simulink library "inp"  (R2021b)
settings: Solver=VariableStepAuto  StartTime=0.0  StopTime=10.0  RelTol=1e-3
undefined symbols (not defined in the file): C_TASK_5MS_S, FALSE, KINP_AcoreReadyToSlp_flg_ovrdflg, KINP_AcoreReadyToSlp_flg_ovrdval, KINP_AllowMovThd_OTA_enum_ovrdflg, KINP_AllowMovThd_OTA_enum_ovrdval, KINP_APSAngleTarget_Deg_ovrdflg, KINP_APSAngleTarget_Deg_ovrdval, KINP_APSDecReq_mps2_ovrdflg, KINP_APSDecReq_mps2_ovrdval, KINP_APSDecReqA_flg_ovrdflg, KINP_APSDecReqA_flg_ovrdval, KINP_APSDFLL_cm_ovrdflg, KINP_APSDFLL_cm_ovrdval, KINP_APSDFLR_cm_ovrdflg, KINP_APSDFLR_cm_ovrdval, KINP_APSDRLL_cm_ovrdflg, KINP_APSDRLL_cm_ovrdval, KINP_APSDRLR_cm_ovrdflg, KINP_APSDRLR_cm_ovrdval, KINP_APSExitCondition_enum_ovrdflg, KINP_APSExitCondition_enum_ovrdval, KINP_APSHWVer_enum_ovrdflg, KINP_APSHWVer_enum_ovrdval, KINP_APSProgressPCT_pct_ovrdflg, KINP_APSProgressPCT_pct_ovrdval, KINP_APSReq_enum_ovrdflg, KINP_APSReq_enum_ovrdval, KINP_APSRQDisplay_enum_ovrdflg, KINP_APSRQDisplay_enum_ovrdval, KINP_APSRqEPASCtrl_flg_ovrdflg, KINP_APSRqEPASCtrl_flg_ovrdval, KINP_APSShiftPosnReq_enum_ovrdval, KINP_APSShiftPosnReq_enum_ovrflg, KINP_APSSpeedCMD_kph_ovrdval, KINP_APSSpeedCMD_kph_ovrflg, KINP_APSStaSystem_enum_ovrdflg, KINP_APSStaSystem_enum_ovrdval, KINP_APSSWVer_enum_ovrdflg, KINP_APSSWVer_enum_ovrdval, KINP_APSVMCReqA_flg_ovrdval, KINP_APSVMCReqA_flg_ovrflg, KINP_APSVRqEPASCtrl_flg_ovrdflg, KINP_APSVRqEPASCtrl_flg_ovrdval, KINP_AuxBattVolmV_mV_ovrdflg, KINP_AuxBattVolmV_mV_ovrdval, KINP_CAASSta_enum_ovrdflg, KINP_CAASSta_enum_ovrdval, KINP_CAASVMCReqA_flg_ovrdval, KINP_CAASVMCReqA_flg_ovrflg, KINP_Chime_enum_ovrdflg, KINP_Chime_enum_ovrdval, KINP_ClearDTCcmd_flg_ovrdflg, KINP_ClearDTCcmd_flg_ovrdval, KINP_EvccAplusPwrUpReq_flg_ovrdflg, KINP_EvccAplusPwrUpReq_flg_ovrdval, KINP_LFID_raw_ovrdval, KINP_LFID_raw_ovrflg, KINP_LRID_raw_ovrdval, KINP_MemOffsetAccX_raw16_ovrdflg ... (+118)
libraries: FVT_lib x595, hcu_lib x1
(part 26 of 27)

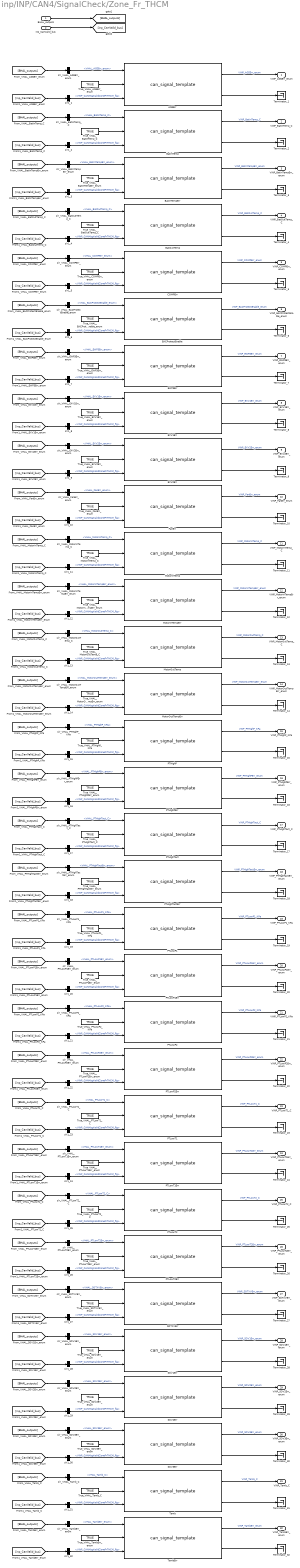
== system inp/INP/CAN4/SignalCheck/Zone_Fr_THCM ==
  BHAL_outputs : Inport
  inp_CanValid_bus : Inport  Port=2
  AGSErr : FVT_lib/inp/can_signal_template  SystemSampleTime=-1  VariantActivationTime=update diagram  Latency=0  AutoFrameSizeCalculation=off
      link override defval: Value=KINP_AGSErr_enum_defval
      link override fftdec: Value=KINP_AGSErr_enum_fftdec
      link override fftinc: Value=KINP_AGSErr_enum_fftinc
      link override fftlim: Value=KINP_AGSErr_enum_fftlim
      link override invalid: Value=KINP_AGSErr_enum_invalid
      link override ovrdflg: Value=KINP_AGSErr_enum_ovrdflg
      link override ovrdval: Value=KINP_AGSErr_enum_ovrdval
      link override setvalid: Value=KINP_AGSErr_enum_setvalid
      link override srvcflg: Value=KINP_AGSErr_enum_srvcflg
      link override srvcval: Value=KINP_AGSErr_enum_srvcval
  BatInTemp : FVT_lib/inp/can_signal_template  SystemSampleTime=-1  VariantActivationTime=update diagram  Latency=0  AutoFrameSizeCalculation=off
      link override defval: Value=KINP_BatInTemp_C_defval
      link override fftdec: Value=KINP_BatInTemp_C_fftdec
      link override fftinc: Value=KINP_BatInTemp_C_fftinc
      link override fftlim: Value=KINP_BatInTemp_C_fftlim
      link override invalid: Value=KINP_BatInTemp_C_invalid
      link override ovrdflg: Value=KINP_BatInTemp_C_ovrdflg
      link override ovrdval: Value=KINP_BatInTemp_C_ovrdval
      link override setvalid: Value=KINP_BatInTemp_C_setvalid
      link override srvcflg: Value=KINP_BatInTemp_C_srvcflg
      link override srvcval: Value=KINP_BatInTemp_C_srvcval
  BatInTempErr : FVT_lib/inp/can_signal_template  SystemSampleTime=-1  VariantActivationTime=update diagram  Latency=0  AutoFrameSizeCalculation=off
      link override defval: Value=KINP_BatInTempErr_enum_defval
      link override fftdec: Value=KINP_BatInTempErr_enum_fftdec
      link override fftinc: Value=KINP_BatInTempErr_enum_fftinc
      link override fftlim: Value=KINP_BatInTempErr_enum_fftlim
      link override invalid: Value=KINP_BatInTempErr_enum_invalid
      link override ovrdflg: Value=KINP_BatInTempErr_enum_ovrdflg
      link override ovrdval: Value=KINP_BatInTempErr_enum_ovrdval
      link override setvalid: Value=KINP_BatInTempErr_enum_setvalid
      link override srvcflg: Value=KINP_BatInTempErr_enum_srvcflg
      link override srvcval: Value=KINP_BatInTempErr_enum_srvcval
  BatOutTemp : FVT_lib/inp/can_signal_template  SystemSampleTime=-1  VariantActivationTime=update diagram  Latency=0  AutoFrameSizeCalculation=off
      link override defval: Value=KINP_BatOutTemp_C_defval
      link override fftdec: Value=KINP_BatOutTemp_C_fftdec
      link override fftinc: Value=KINP_BatOutTemp_C_fftinc
      link override fftlim: Value=KINP_BatOutTemp_C_fftlim
      link override invalid: Value=KINP_BatOutTemp_C_invalid
      link override ovrdflg: Value=KINP_BatOutTemp_C_ovrdflg
      link override ovrdval: Value=KINP_BatOutTemp_C_ovrdval
      link override setvalid: Value=KINP_BatOutTemp_C_setvalid
      link override srvcflg: Value=KINP_BatOutTemp_C_srvcflg
      link override srvcval: Value=KINP_BatOutTemp_C_srvcval
  COMPErr : FVT_lib/inp/can_signal_template  SystemSampleTime=-1  VariantActivationTime=update diagram  Latency=0  AutoFrameSizeCalculation=off
      link override defval: Value=KINP_COMPErr_enum_defval
      link override fftdec: Value=KINP_COMPErr_enum_fftdec
      link override fftinc: Value=KINP_COMPErr_enum_fftinc
      link override fftlim: Value=KINP_COMPErr_enum_fftlim
      link override invalid: Value=KINP_COMPErr_enum_invalid
      link override ovrdflg: Value=KINP_COMPErr_enum_ovrdflg
      link override ovrdval: Value=KINP_COMPErr_enum_ovrdval
      link override setvalid: Value=KINP_COMPErr_enum_setvalid
      link override srvcflg: Value=KINP_COMPErr_enum_srvcflg
      link override srvcval: Value=KINP_COMPErr_enum_srvcval
  EACProtectEnable : FVT_lib/inp/can_signal_template  SystemSampleTime=-1  VariantActivationTime=update diagram  Latency=0  AutoFrameSizeCalculation=off
      link override defval: Value=KINP_EACProtectEnable_enum_defval
      link override fftdec: Value=KINP_EACProtectEnable_enum_fftdec
      link override fftinc: Value=KINP_EACProtectEnable_enum_fftinc
      link override fftlim: Value=KINP_EACProtectEnable_enum_fftlim
      link override invalid: Value=KINP_EACProtectEnable_enum_invalid
      link override ovrdflg: Value=KINP_EACProtectEnable_enum_ovrdflg
      link override ovrdval: Value=KINP_EACProtectEnable_enum_ovrdval
      link override setvalid: Value=KINP_EACProtectEnable_enum_setvalid
      link override srvcflg: Value=KINP_EACProtectEnable_enum_srvcflg
      link override srvcval: Value=KINP_EACProtectEnable_enum_srvcval
  EWP3Err : FVT_lib/inp/can_signal_template  SystemSampleTime=-1  VariantActivationTime=update diagram  Latency=0  AutoFrameSizeCalculation=off
      link override defval: Value=KINP_EWP3Err_enum_defval
      link override fftdec: Value=KINP_EWP3Err_enum_fftdec
      link override fftinc: Value=KINP_EWP3Err_enum_fftinc
      link override fftlim: Value=KINP_EWP3Err_enum_fftlim
      link override invalid: Value=KINP_EWP3Err_enum_invalid
      link override ovrdflg: Value=KINP_EWP3Err_enum_ovrdflg
      link override ovrdval: Value=KINP_EWP3Err_enum_ovrdval
      link override setvalid: Value=KINP_EWP3Err_enum_setvalid
      link override srvcflg: Value=KINP_EWP3Err_enum_srvcflg
      link override srvcval: Value=KINP_EWP3Err_enum_srvcval
  EXV1Err : FVT_lib/inp/can_signal_template  SystemSampleTime=-1  VariantActivationTime=update diagram  Latency=0  AutoFrameSizeCalculation=off
      link override defval: Value=KINP_EXV1Err_enum_defval
      link override fftdec: Value=KINP_EXV1Err_enum_fftdec
      link override fftinc: Value=KINP_EXV1Err_enum_fftinc
      link override fftlim: Value=KINP_EXV1Err_enum_fftlim
      link override invalid: Value=KINP_EXV1Err_enum_invalid
      link override ovrdflg: Value=KINP_EXV1Err_enum_ovrdflg
      link override ovrdval: Value=KINP_EXV1Err_enum_ovrdval
      link override setvalid: Value=KINP_EXV1Err_enum_setvalid
      link override srvcflg: Value=KINP_EXV1Err_enum_srvcflg
      link override srvcval: Value=KINP_EXV1Err_enum_srvcval
  EXV2Err : FVT_lib/inp/can_signal_template  SystemSampleTime=-1  VariantActivationTime=update diagram  Latency=0  AutoFrameSizeCalculation=off
      link override defval: Value=KINP_EXV2Err_enum_defval
      link override fftdec: Value=KINP_EXV2Err_enum_fftdec
      link override fftinc: Value=KINP_EXV2Err_enum_fftinc
      link override fftlim: Value=KINP_EXV2Err_enum_fftlim
      link override invalid: Value=KINP_EXV2Err_enum_invalid
      link override ovrdflg: Value=KINP_EXV2Err_enum_ovrdflg
      link override ovrdval: Value=KINP_EXV2Err_enum_ovrdval
      link override setvalid: Value=KINP_EXV2Err_enum_setvalid
      link override srvcflg: Value=KINP_EXV2Err_enum_srvcflg
      link override srvcval: Value=KINP_EXV2Err_enum_srvcval
  FanErr : FVT_lib/inp/can_signal_template  SystemSampleTime=-1  VariantActivationTime=update diagram  Latency=0  AutoFrameSizeCalculation=off
      link override defval: Value=KINP_FanErr_enum_defval
      link override fftdec: Value=KINP_FanErr_enum_fftdec
      link override fftinc: Value=KINP_FanErr_enum_fftinc
      link override fftlim: Value=KINP_FanErr_enum_fftlim
      link override invalid: Value=KINP_FanErr_enum_invalid
      link override ovrdflg: Value=KINP_FanErr_enum_ovrdflg
      link override ovrdval: Value=KINP_FanErr_enum_ovrdval
      link override setvalid: Value=KINP_FanErr_enum_setvalid
      link override srvcflg: Value=KINP_FanErr_enum_srvcflg
      link override srvcval: Value=KINP_FanErr_enum_srvcval
  MotorInTemp : FVT_lib/inp/can_signal_template  SystemSampleTime=-1  VariantActivationTime=update diagram  Latency=0  AutoFrameSizeCalculation=off
      link override defval: Value=KINP_MotorInTemp_C_defval
      link override fftdec: Value=KINP_MotorInTemp_C_fftdec
      link override fftinc: Value=KINP_MotorInTemp_C_fftinc
      link override fftlim: Value=KINP_MotorInTemp_C_fftlim
      link override invalid: Value=KINP_MotorInTemp_C_invalid
      link override ovrdflg: Value=KINP_MotorInTemp_C_ovrdflg
      link override ovrdval: Value=KINP_MotorInTemp_C_ovrdval
      link override setvalid: Value=KINP_MotorInTemp_C_setvalid
      link override srvcflg: Value=KINP_MotorInTemp_C_srvcflg
      link override srvcval: Value=KINP_MotorInTemp_C_srvcval
  MotorInTempErr : FVT_lib/inp/can_signal_template  SystemSampleTime=-1  VariantActivationTime=update diagram  Latency=0  AutoFrameSizeCalculation=off
      link override defval: Value=KINP_MotorInTempErr_enum_defval
      link override fftdec: Value=KINP_MotorInTempErr_enum_fftdec
      link override fftinc: Value=KINP_MotorInTempErr_enum_fftinc
      link override fftlim: Value=KINP_MotorInTempErr_enum_fftlim
      link override invalid: Value=KINP_MotorInTempErr_enum_invalid
      link override ovrdflg: Value=KINP_MotorInTempErr_enum_ovrdflg
      link override ovrdval: Value=KINP_MotorInTempErr_enum_ovrdval
      link override setvalid: Value=KINP_MotorInTempErr_enum_setvalid
      link override srvcflg: Value=KINP_MotorInTempErr_enum_srvcflg
      link override srvcval: Value=KINP_MotorInTempErr_enum_srvcval
  MotorOutTemp : FVT_lib/inp/can_signal_template  SystemSampleTime=-1  VariantActivationTime=update diagram  Latency=0  AutoFrameSizeCalculation=off
      link override defval: Value=KINP_MotorOutTemp_C_defval
      link override fftdec: Value=KINP_MotorOutTemp_C_fftdec
      link override fftinc: Value=KINP_MotorOutTemp_C_fftinc
      link override fftlim: Value=KINP_MotorOutTemp_C_fftlim
      link override invalid: Value=KINP_MotorOutTemp_C_invalid
      link override ovrdflg: Value=KINP_MotorOutTemp_C_ovrdflg
      link override ovrdval: Value=KINP_MotorOutTemp_C_ovrdval
      link override setvalid: Value=KINP_MotorOutTemp_C_setvalid
      link override srvcflg: Value=KINP_MotorOutTemp_C_srvcflg
      link override srvcval: Value=KINP_MotorOutTemp_C_srvcval
  MotorOutTempErr : FVT_lib/inp/can_signal_template  SystemSampleTime=-1  VariantActivationTime=update diagram  Latency=0  AutoFrameSizeCalculation=off
      link override defval: Value=KINP_MotorOutTempErr_enum_defval
      link override fftdec: Value=KINP_MotorOutTempErr_enum_fftdec
      link override fftinc: Value=KINP_MotorOutTempErr_enum_fftinc
      link override fftlim: Value=KINP_MotorOutTempErr_enum_fftlim
      link override invalid: Value=KINP_MotorOutTempErr_enum_invalid
      link override ovrdflg: Value=KINP_MotorOutTempErr_enum_ovrdflg
      link override ovrdval: Value=KINP_MotorOutTempErr_enum_ovrdval
      link override setvalid: Value=KINP_MotorOutTempErr_enum_setvalid
      link override srvcflg: Value=KINP_MotorOutTempErr_enum_srvcflg
      link override srvcval: Value=KINP_MotorOutTempErr_enum_srvcval
  PTHighP : FVT_lib/inp/can_signal_template  SystemSampleTime=-1  VariantActivationTime=update diagram  Latency=0  AutoFrameSizeCalculation=off
      link override defval: Value=KINP_PTHighP_KPa_defval
      link override fftdec: Value=KINP_PTHighP_KPa_fftdec
      link override fftinc: Value=KINP_PTHighP_KPa_fftinc
      link override fftlim: Value=KINP_PTHighP_KPa_fftlim
      link override invalid: Value=KINP_PTHighP_KPa_invalid
      link override ovrdflg: Value=KINP_PTHighP_KPa_ovrdflg
      link override ovrdval: Value=KINP_PTHighP_KPa_ovrdval
      link override setvalid: Value=KINP_PTHighP_KPa_setvalid
      link override srvcflg: Value=KINP_PTHighP_KPa_srvcflg
      link override srvcval: Value=KINP_PTHighP_KPa_srvcval
  PTHighPErr : FVT_lib/inp/can_signal_template  SystemSampleTime=-1  VariantActivationTime=update diagram  Latency=0  AutoFrameSizeCalculation=off
      link override defval: Value=KINP_PTHighPErr_enum_defval
      link override fftdec: Value=KINP_PTHighPErr_enum_fftdec
      link override fftinc: Value=KINP_PTHighPErr_enum_fftinc
      link override fftlim: Value=KINP_PTHighPErr_enum_fftlim
      link override invalid: Value=KINP_PTHighPErr_enum_invalid
      link override ovrdflg: Value=KINP_PTHighPErr_enum_ovrdflg
      link override ovrdval: Value=KINP_PTHighPErr_enum_ovrdval
      link override setvalid: Value=KINP_PTHighPErr_enum_setvalid
      link override srvcflg: Value=KINP_PTHighPErr_enum_srvcflg
      link override srvcval: Value=KINP_PTHighPErr_enum_srvcval
  PTHighTact : FVT_lib/inp/can_signal_template  SystemSampleTime=-1  VariantActivationTime=update diagram  Latency=0  AutoFrameSizeCalculation=off
      link override defval: Value=KINP_PTHighTact_C_defval
      link override fftdec: Value=KINP_PTHighTact_C_fftdec
      link override fftinc: Value=KINP_PTHighTact_C_fftinc
      link override fftlim: Value=KINP_PTHighTact_C_fftlim
      link override invalid: Value=KINP_PTHighTact_C_invalid
      link override ovrdflg: Value=KINP_PTHighTact_C_ovrdflg
      link override ovrdval: Value=KINP_PTHighTact_C_ovrdval
      link override setvalid: Value=KINP_PTHighTact_C_setvalid
      link override srvcflg: Value=KINP_PTHighTact_C_srvcflg
      link override srvcval: Value=KINP_PTHighTact_C_srvcval
  PTHighTactErr : FVT_lib/inp/can_signal_template  SystemSampleTime=-1  VariantActivationTime=update diagram  Latency=0  AutoFrameSizeCalculation=off
      link override defval: Value=KINP_PTHighTactErr_enum_defval
      link override fftdec: Value=KINP_PTHighTactErr_enum_fftdec
      link override fftinc: Value=KINP_PTHighTactErr_enum_fftinc
      link override fftlim: Value=KINP_PTHighTactErr_enum_fftlim
      link override invalid: Value=KINP_PTHighTactErr_enum_invalid
      link override ovrdflg: Value=KINP_PTHighTactErr_enum_ovrdflg
      link override ovrdval: Value=KINP_PTHighTactErr_enum_ovrdval
      link override setvalid: Value=KINP_PTHighTactErr_enum_setvalid
      link override srvcflg: Value=KINP_PTHighTactErr_enum_srvcflg
      link override srvcval: Value=KINP_PTHighTactErr_enum_srvcval
  PTLowP1 : FVT_lib/inp/can_signal_template  SystemSampleTime=-1  VariantActivationTime=update diagram  Latency=0  AutoFrameSizeCalculation=off
      link override defval: Value=KINP_PTLowP1_KPa_defval
      link override fftdec: Value=KINP_PTLowP1_KPa_fftdec
      link override fftinc: Value=KINP_PTLowP1_KPa_fftinc
      link override fftlim: Value=KINP_PTLowP1_KPa_fftlim
      link override invalid: Value=KINP_PTLowP1_KPa_invalid
      link override ovrdflg: Value=KINP_PTLowP1_KPa_ovrdflg
      link override ovrdval: Value=KINP_PTLowP1_KPa_ovrdval
      link override setvalid: Value=KINP_PTLowP1_KPa_setvalid
      link override srvcflg: Value=KINP_PTLowP1_KPa_srvcflg
      link override srvcval: Value=KINP_PTLowP1_KPa_srvcval
  PTLowP1Err : FVT_lib/inp/can_signal_template  SystemSampleTime=-1  VariantActivationTime=update diagram  Latency=0  AutoFrameSizeCalculation=off
      link override defval: Value=KINP_PTLowP1Err_enum_defval
      link override fftdec: Value=KINP_PTLowP1Err_enum_fftdec
      link override fftinc: Value=KINP_PTLowP1Err_enum_fftinc
      link override fftlim: Value=KINP_PTLowP1Err_enum_fftlim
      link override invalid: Value=KINP_PTLowP1Err_enum_invalid
      link override ovrdflg: Value=KINP_PTLowP1Err_enum_ovrdflg
      link override ovrdval: Value=KINP_PTLowP1Err_enum_ovrdval
      link override setvalid: Value=KINP_PTLowP1Err_enum_setvalid
      link override srvcflg: Value=KINP_PTLowP1Err_enum_srvcflg
      link override srvcval: Value=KINP_PTLowP1Err_enum_srvcval
  PTLowP2 : FVT_lib/inp/can_signal_template  SystemSampleTime=-1  VariantActivationTime=update diagram  Latency=0  AutoFrameSizeCalculation=off
      link override defval: Value=KINP_PTLowP2_KPa_defval
      link override fftdec: Value=KINP_PTLowP2_KPa_fftdec
      link override fftinc: Value=KINP_PTLowP2_KPa_fftinc
      link override fftlim: Value=KINP_PTLowP2_KPa_fftlim
      link override invalid: Value=KINP_PTLowP2_KPa_invalid
      link override ovrdflg: Value=KINP_PTLowP2_KPa_ovrdflg
      link override ovrdval: Value=KINP_PTLowP2_KPa_ovrdval
      link override setvalid: Value=KINP_PTLowP2_KPa_setvalid
      link override srvcflg: Value=KINP_PTLowP2_KPa_srvcflg
      link override srvcval: Value=KINP_PTLowP2_KPa_srvcval
  PTLowP2Err : FVT_lib/inp/can_signal_template  SystemSampleTime=-1  VariantActivationTime=update diagram  Latency=0  AutoFrameSizeCalculation=off
      link override defval: Value=KINP_PTLowP2Err_enum_defval
      link override fftdec: Value=KINP_PTLowP2Err_enum_fftdec
      link override fftinc: Value=KINP_PTLowP2Err_enum_fftinc
      link override fftlim: Value=KINP_PTLowP2Err_enum_fftlim
      link override invalid: Value=KINP_PTLowP2Err_enum_invalid
      link override ovrdflg: Value=KINP_PTLowP2Err_enum_ovrdflg
      link override ovrdval: Value=KINP_PTLowP2Err_enum_ovrdval
      link override setvalid: Value=KINP_PTLowP2Err_enum_setvalid
      link override srvcflg: Value=KINP_PTLowP2Err_enum_srvcflg
      link override srvcval: Value=KINP_PTLowP2Err_enum_srvcval
  PTLowT1 : FVT_lib/inp/can_signal_template  SystemSampleTime=-1  VariantActivationTime=update diagram  Latency=0  AutoFrameSizeCalculation=off
      link override defval: Value=KINP_PTLowT1_C_defval
      link override fftdec: Value=KINP_PTLowT1_C_fftdec
      link override fftinc: Value=KINP_PTLowT1_C_fftinc
      link override fftlim: Value=KINP_PTLowT1_C_fftlim
      link override invalid: Value=KINP_PTLowT1_C_invalid
      link override ovrdflg: Value=KINP_PTLowT1_C_ovrdflg
      link override ovrdval: Value=KINP_PTLowT1_C_ovrdval
      link override setvalid: Value=KINP_PTLowT1_C_setvalid
      link override srvcflg: Value=KINP_PTLowT1_C_srvcflg
      link override srvcval: Value=KINP_PTLowT1_C_srvcval
  PTLowT1Err : FVT_lib/inp/can_signal_template  SystemSampleTime=-1  VariantActivationTime=update diagram  Latency=0  AutoFrameSizeCalculation=off
      link override defval: Value=KINP_PTLowT1Err_enum_defval
      link override fftdec: Value=KINP_PTLowT1Err_enum_fftdec
      link override fftinc: Value=KINP_PTLowT1Err_enum_fftinc
      link override fftlim: Value=KINP_PTLowT1Err_enum_fftlim
      link override invalid: Value=KINP_PTLowT1Err_enum_invalid
      link override ovrdflg: Value=KINP_PTLowT1Err_enum_ovrdflg
      link override ovrdval: Value=KINP_PTLowT1Err_enum_ovrdval
      link override setvalid: Value=KINP_PTLowT1Err_enum_setvalid
      link override srvcflg: Value=KINP_PTLowT1Err_enum_srvcflg
      link override srvcval: Value=KINP_PTLowT1Err_enum_srvcval
  PTLowT2 : FVT_lib/inp/can_signal_template  SystemSampleTime=-1  VariantActivationTime=update diagram  Latency=0  AutoFrameSizeCalculation=off
      link override defval: Value=KINP_PTLowT2_C_defval
      link override fftdec: Value=KINP_PTLowT2_C_fftdec
      link override fftinc: Value=KINP_PTLowT2_C_fftinc
      link override fftlim: Value=KINP_PTLowT2_C_fftlim
      link override invalid: Value=KINP_PTLowT2_C_invalid
      link override ovrdflg: Value=KINP_PTLowT2_C_ovrdflg
      link override ovrdval: Value=KINP_PTLowT2_C_ovrdval
      link override setvalid: Value=KINP_PTLowT2_C_setvalid
      link override srvcflg: Value=KINP_PTLowT2_C_srvcflg
      link override srvcval: Value=KINP_PTLowT2_C_srvcval
  PTLowT2Err : FVT_lib/inp/can_signal_template  SystemSampleTime=-1  VariantActivationTime=update diagram  Latency=0  AutoFrameSizeCalculation=off
      link override defval: Value=KINP_PTLowT2Err_enum_defval
      link override fftdec: Value=KINP_PTLowT2Err_enum_fftdec
      link override fftinc: Value=KINP_PTLowT2Err_enum_fftinc
      link override fftlim: Value=KINP_PTLowT2Err_enum_fftlim
      link override invalid: Value=KINP_PTLowT2Err_enum_invalid
      link override ovrdflg: Value=KINP_PTLowT2Err_enum_ovrdflg
      link override ovrdval: Value=KINP_PTLowT2Err_enum_ovrdval
      link override setvalid: Value=KINP_PTLowT2Err_enum_setvalid
      link override srvcflg: Value=KINP_PTLowT2Err_enum_srvcflg
      link override srvcval: Value=KINP_PTLowT2Err_enum_srvcval
  SOTXVErr : FVT_lib/inp/can_signal_template  SystemSampleTime=-1  VariantActivationTime=update diagram  Latency=0  AutoFrameSizeCalculation=off
      link override defval: Value=KINP_SOTXVErr_enum_defval
      link override fftdec: Value=KINP_SOTXVErr_enum_fftdec
      link override fftinc: Value=KINP_SOTXVErr_enum_fftinc
      link override fftlim: Value=KINP_SOTXVErr_enum_fftlim
      link override invalid: Value=KINP_SOTXVErr_enum_invalid
      link override ovrdflg: Value=KINP_SOTXVErr_enum_ovrdflg
      link override ovrdval: Value=KINP_SOTXVErr_enum_ovrdval
      link override setvalid: Value=KINP_SOTXVErr_enum_setvalid
      link override srvcflg: Value=KINP_SOTXVErr_enum_srvcflg
      link override srvcval: Value=KINP_SOTXVErr_enum_srvcval
  SOV1Err : FVT_lib/inp/can_signal_template  SystemSampleTime=-1  VariantActivationTime=update diagram  Latency=0  AutoFrameSizeCalculation=off
      link override defval: Value=KINP_SOV1Err_enum_defval
      link override fftdec: Value=KINP_SOV1Err_enum_fftdec
      link override fftinc: Value=KINP_SOV1Err_enum_fftinc
      link override fftlim: Value=KINP_SOV1Err_enum_fftlim
      link override invalid: Value=KINP_SOV1Err_enum_invalid
      link override ovrdflg: Value=KINP_SOV1Err_enum_ovrdflg
      link override ovrdval: Value=KINP_SOV1Err_enum_ovrdval
      link override setvalid: Value=KINP_SOV1Err_enum_setvalid
      link override srvcflg: Value=KINP_SOV1Err_enum_srvcflg
      link override srvcval: Value=KINP_SOV1Err_enum_srvcval
  SOV2Err : FVT_lib/inp/can_signal_template  SystemSampleTime=-1  VariantActivationTime=update diagram  Latency=0  AutoFrameSizeCalculation=off
      link override defval: Value=KINP_SOV2Err_enum_defval
      link override fftdec: Value=KINP_SOV2Err_enum_fftdec
      link override fftinc: Value=KINP_SOV2Err_enum_fftinc
      link override fftlim: Value=KINP_SOV2Err_enum_fftlim
      link override invalid: Value=KINP_SOV2Err_enum_invalid
      link override ovrdflg: Value=KINP_SOV2Err_enum_ovrdflg
      link override ovrdval: Value=KINP_SOV2Err_enum_ovrdval
      link override setvalid: Value=KINP_SOV2Err_enum_setvalid
      link override srvcflg: Value=KINP_SOV2Err_enum_srvcflg
      link override srvcval: Value=KINP_SOV2Err_enum_srvcval
  SOV3Err : FVT_lib/inp/can_signal_template  SystemSampleTime=-1  VariantActivationTime=update diagram  Latency=0  AutoFrameSizeCalculation=off
      link override defval: Value=KINP_SOV3Err_enum_defval
      link override fftdec: Value=KINP_SOV3Err_enum_fftdec
      link override fftinc: Value=KINP_SOV3Err_enum_fftinc
      link override fftlim: Value=KINP_SOV3Err_enum_fftlim
      link override invalid: Value=KINP_SOV3Err_enum_invalid
      link override ovrdflg: Value=KINP_SOV3Err_enum_ovrdflg
      link override ovrdval: Value=KINP_SOV3Err_enum_ovrdval
      link override setvalid: Value=KINP_SOV3Err_enum_setvalid
      link override srvcflg: Value=KINP_SOV3Err_enum_srvcflg
      link override srvcval: Value=KINP_SOV3Err_enum_srvcval
  Tamb : FVT_lib/inp/can_signal_template  SystemSampleTime=-1  VariantActivationTime=update diagram  Latency=0  AutoFrameSizeCalculation=off
      link override defval: Value=KINP_Tamb_C_defval
      link override fftdec: Value=KINP_Tamb_C_fftdec
      link override fftinc: Value=KINP_Tamb_C_fftinc
      link override fftlim: Value=KINP_Tamb_C_fftlim
      link override invalid: Value=KINP_Tamb_C_invalid
      link override ovrdflg: Value=KINP_Tamb_C_ovrdflg
      link override ovrdval: Value=KINP_Tamb_C_ovrdval
      link override setvalid: Value=KINP_Tamb_C_setvalid
      link override srvcflg: Value=KINP_Tamb_C_srvcflg
      link override srvcval: Value=KINP_Tamb_C_srvcval
  TambErr : FVT_lib/inp/can_signal_template  SystemSampleTime=-1  VariantActivationTime=update diagram  Latency=0  AutoFrameSizeCalculation=off
      link override defval: Value=KINP_TambErr_enum_defval
      link override fftdec: Value=KINP_TambErr_enum_fftdec
      link override fftinc: Value=KINP_TambErr_enum_fftinc
      link override fftlim: Value=KINP_TambErr_enum_fftlim
      link override invalid: Value=KINP_TambErr_enum_invalid
      link override ovrdflg: Value=KINP_TambErr_enum_ovrdflg
      link override ovrdval: Value=KINP_TambErr_enum_ovrdval
      link override setvalid: Value=KINP_TambErr_enum_setvalid
      link override srvcflg: Value=KINP_TambErr_enum_srvcflg
      link override srvcval: Value=KINP_TambErr_enum_srvcval
  Terminator_{1..32} (32 alike) : Terminator
  True_VHAL_AGSErr_enum : Constant  Value=TRUE  OutDataTypeStr=boolean
  True_VHAL_BatInTempErr_enum : Constant  Value=TRUE  OutDataTypeStr=boolean
  True_VHAL_BatInTemp_C : Constant  Value=TRUE  OutDataTypeStr=boolean
  True_VHAL_BatOutTemp_C : Constant  Value=TRUE  OutDataTypeStr=boolean
  True_VHAL_COMPErr_enum : Constant  Value=TRUE  OutDataTypeStr=boolean
  True_VHAL_EACProtectEnable_enum : Constant  Value=TRUE  OutDataTypeStr=boolean
  True_VHAL_EWP3Err_enum : Constant  Value=TRUE  OutDataTypeStr=boolean
  True_VHAL_EXV1Err_enum : Constant  Value=TRUE  OutDataTypeStr=boolean
  True_VHAL_EXV2Err_enum : Constant  Value=TRUE  OutDataTypeStr=boolean
  True_VHAL_FanErr_enum : Constant  Value=TRUE  OutDataTypeStr=boolean
  True_VHAL_MotorInTempErr_enum : Constant  Value=TRUE  OutDataTypeStr=boolean
  True_VHAL_MotorInTemp_C : Constant  Value=TRUE  OutDataTypeStr=boolean
  True_VHAL_MotorOutTempErr_enum : Constant  Value=TRUE  OutDataTypeStr=boolean
  True_VHAL_MotorOutTemp_C : Constant  Value=TRUE  OutDataTypeStr=boolean
  True_VHAL_PTHighPErr_enum : Constant  Value=TRUE  OutDataTypeStr=boolean
  True_VHAL_PTHighP_KPa : Constant  Value=TRUE  OutDataTypeStr=boolean
  True_VHAL_PTHighTactErr_enum : Constant  Value=TRUE  OutDataTypeStr=boolean
  True_VHAL_PTHighTact_C : Constant  Value=TRUE  OutDataTypeStr=boolean
  True_VHAL_PTLowP1Err_enum : Constant  Value=TRUE  OutDataTypeStr=boolean
  True_VHAL_PTLowP1_KPa : Constant  Value=TRUE  OutDataTypeStr=boolean
  True_VHAL_PTLowP2Err_enum : Constant  Value=TRUE  OutDataTypeStr=boolean
  True_VHAL_PTLowP2_KPa : Constant  Value=TRUE  OutDataTypeStr=boolean
  True_VHAL_PTLowT1Err_enum : Constant  Value=TRUE  OutDataTypeStr=boolean
  True_VHAL_PTLowT1_C : Constant  Value=TRUE  OutDataTypeStr=boolean
  True_VHAL_PTLowT2Err_enum : Constant  Value=TRUE  OutDataTypeStr=boolean
  True_VHAL_PTLowT2_C : Constant  Value=TRUE  OutDataTypeStr=boolean
  True_VHAL_SOTXVErr_enum : Constant  Value=TRUE  OutDataTypeStr=boolean
  True_VHAL_SOV1Err_enum : Constant  Value=TRUE  OutDataTypeStr=boolean
  True_VHAL_SOV2Err_enum : Constant  Value=TRUE  OutDataTypeStr=boolean
  True_VHAL_SOV3Err_enum : Constant  Value=TRUE  OutDataTypeStr=boolean
  True_VHAL_TambErr_enum : Constant  Value=TRUE  OutDataTypeStr=boolean
  True_VHAL_Tamb_C : Constant  Value=TRUE  OutDataTypeStr=boolean
  slr1_{1..32} (32 alike) : BusSelector  OutputSignals=VINP_CANMsgValidZoneFrTHCM_flg
  slr_VHAL_AGSErr_enum : BusSelector  OutputSignals=VHAL_AGSErr_enum
  slr_VHAL_BatInTempErr_enum : BusSelector  OutputSignals=VHAL_BatInTempErr_enum
  slr_VHAL_BatInTemp_C : BusSelector  OutputSignals=VHAL_BatInTemp_C
  slr_VHAL_BatOutTemp_C : BusSelector  OutputSignals=VHAL_BatOutTemp_C
  slr_VHAL_COMPErr_enum : BusSelector  OutputSignals=VHAL_COMPErr_enum
  slr_VHAL_EACProtectEnable_enum : BusSelector  OutputSignals=VHAL_EACProtectEnable_enum
  slr_VHAL_EWP3Err_enum : BusSelector  OutputSignals=VHAL_EWP3Err_enum
  slr_VHAL_EXV1Err_enum : BusSelector  OutputSignals=VHAL_EXV1Err_enum
  slr_VHAL_EXV2Err_enum : BusSelector  OutputSignals=VHAL_EXV2Err_enum
  slr_VHAL_FanErr_enum : BusSelector  OutputSignals=VHAL_FanErr_enum
  slr_VHAL_MotorInTempErr_enum : BusSelector  OutputSignals=VHAL_MotorInTempErr_enum
  slr_VHAL_MotorInTemp_C : BusSelector  OutputSignals=VHAL_MotorInTemp_C
  slr_VHAL_MotorOutTempErr_enum : BusSelector  OutputSignals=VHAL_MotorOutTempErr_enum
  slr_VHAL_MotorOutTemp_C : BusSelector  OutputSignals=VHAL_MotorOutTemp_C
  slr_VHAL_PTHighPErr_enum : BusSelector  OutputSignals=VHAL_PTHighPErr_enum
  slr_VHAL_PTHighP_KPa : BusSelector  OutputSignals=VHAL_PTHighP_KPa
  slr_VHAL_PTHighTactErr_enum : BusSelector  OutputSignals=VHAL_PTHighTactErr_enum
  slr_VHAL_PTHighTact_C : BusSelector  OutputSignals=VHAL_PTHighTact_C
  slr_VHAL_PTLowP1Err_enum : BusSelector  OutputSignals=VHAL_PTLowP1Err_enum
  slr_VHAL_PTLowP1_KPa : BusSelector  OutputSignals=VHAL_PTLowP1_KPa
  slr_VHAL_PTLowP2Err_enum : BusSelector  OutputSignals=VHAL_PTLowP2Err_enum
  slr_VHAL_PTLowP2_KPa : BusSelector  OutputSignals=VHAL_PTLowP2_KPa
  slr_VHAL_PTLowT1Err_enum : BusSelector  OutputSignals=VHAL_PTLowT1Err_enum
  slr_VHAL_PTLowT1_C : BusSelector  OutputSignals=VHAL_PTLowT1_C
  slr_VHAL_PTLowT2Err_enum : BusSelector  OutputSignals=VHAL_PTLowT2Err_enum
  slr_VHAL_PTLowT2_C : BusSelector  OutputSignals=VHAL_PTLowT2_C
  slr_VHAL_SOTXVErr_enum : BusSelector  OutputSignals=VHAL_SOTXVErr_enum
  slr_VHAL_SOV1Err_enum : BusSelector  OutputSignals=VHAL_SOV1Err_enum
  slr_VHAL_SOV2Err_enum : BusSelector  OutputSignals=VHAL_SOV2Err_enum
  slr_VHAL_SOV3Err_enum : BusSelector  OutputSignals=VHAL_SOV3Err_enum
  slr_VHAL_TambErr_enum : BusSelector  OutputSignals=VHAL_TambErr_enum
  slr_VHAL_Tamb_C : BusSelector  OutputSignals=VHAL_Tamb_C
  VINP_AGSErr_enum : Outport
  VINP_BatInTemp_C : Outport  Port=2
  VINP_BatInTempErr_enum : Outport  Port=3
  VINP_BatOutTemp_C : Outport  Port=4
  VINP_COMPErr_enum : Outport  Port=5
  VINP_EACProtectEnable_enum : Outport  Port=6
  VINP_EWP3Err_enum : Outport  Port=7
  VINP_EXV1Err_enum : Outport  Port=8
  VINP_EXV2Err_enum : Outport  Port=9
  VINP_FanErr_enum : Outport  Port=10
  VINP_MotorInTemp_C : Outport  Port=11
  VINP_MotorInTempErr_enum : Outport  Port=12
  VINP_MotorOutTemp_C : Outport  Port=13
  VINP_MotorOutTempErr_enum : Outport  Port=14
  VINP_PTHighP_KPa : Outport  Port=15
  VINP_PTHighPErr_enum : Outport  Port=16
  VINP_PTHighTact_C : Outport  Port=17
  VINP_PTHighTactErr_enum : Outport  Port=18
  VINP_PTLowP1_KPa : Outport  Port=19
  VINP_PTLowP1Err_enum : Outport  Port=20
  VINP_PTLowP2_KPa : Outport  Port=21
  VINP_PTLowP2Err_enum : Outport  Port=22
  VINP_PTLowT1_C : Outport  Port=23
  VINP_PTLowT1Err_enum : Outport  Port=24
  VINP_PTLowT2_C : Outport  Port=25
  VINP_PTLowT2Err_enum : Outport  Port=26
  VINP_SOTXVErr_enum : Outport  Port=27
  VINP_SOV1Err_enum : Outport  Port=28
  VINP_SOV2Err_enum : Outport  Port=29
  VINP_SOV3Err_enum : Outport  Port=30
  VINP_Tamb_C : Outport  Port=31
  VINP_TambErr_enum : Outport  Port=32
  wires:
  BHAL_outputs/1 -> [BHAL_outputs]
  inp_CanValid_bus/1 -> [inp_CanValid_bus]
  [BHAL_outputs] -> slr_VHAL_AGSErr_enum/1
  slr_VHAL_AGSErr_enum/1 -> AGSErr/1  "<VHAL_AGSErr_enum>"
  True_VHAL_AGSErr_enum/1 -> AGSErr/2
  [inp_CanValid_bus] -> slr1_1/1
  slr1_1/1 -> AGSErr/3  "<VINP_CANMsgValidZoneFrTHCM_flg>"
  AGSErr/1 -> VINP_AGSErr_enum/1  "VINP_AGSErr_enum"
  AGSErr/2 -> Terminator_1/1
  [BHAL_outputs] -> slr_VHAL_BatInTemp_C/1
  slr_VHAL_BatInTemp_C/1 -> BatInTemp/1  "<VHAL_BatInTemp_C>"
  True_VHAL_BatInTemp_C/1 -> BatInTemp/2
  [inp_CanValid_bus] -> slr1_2/1
  slr1_2/1 -> BatInTemp/3  "<VINP_CANMsgValidZoneFrTHCM_flg>"
  BatInTemp/1 -> VINP_BatInTemp_C/1  "VINP_BatInTemp_C"
  BatInTemp/2 -> Terminator_2/1
  [BHAL_outputs] -> slr_VHAL_BatInTempErr_enum/1
  slr_VHAL_BatInTempErr_enum/1 -> BatInTempErr/1  "<VHAL_BatInTempErr_enum>"
  True_VHAL_BatInTempErr_enum/1 -> BatInTempErr/2
  [inp_CanValid_bus] -> slr1_3/1
  slr1_3/1 -> BatInTempErr/3  "<VINP_CANMsgValidZoneFrTHCM_flg>"
  BatInTempErr/1 -> VINP_BatInTempErr_enum/1  "VINP_BatInTempErr_enum"
  BatInTempErr/2 -> Terminator_3/1
  [BHAL_outputs] -> slr_VHAL_BatOutTemp_C/1
  slr_VHAL_BatOutTemp_C/1 -> BatOutTemp/1  "<VHAL_BatOutTemp_C>"
  True_VHAL_BatOutTemp_C/1 -> BatOutTemp/2
  [inp_CanValid_bus] -> slr1_4/1
  slr1_4/1 -> BatOutTemp/3  "<VINP_CANMsgValidZoneFrTHCM_flg>"
  BatOutTemp/1 -> VINP_BatOutTemp_C/1  "VINP_BatOutTemp_C"
  BatOutTemp/2 -> Terminator_4/1
  [BHAL_outputs] -> slr_VHAL_COMPErr_enum/1
  slr_VHAL_COMPErr_enum/1 -> COMPErr/1  "<VHAL_COMPErr_enum>"
  True_VHAL_COMPErr_enum/1 -> COMPErr/2
  [inp_CanValid_bus] -> slr1_5/1
  slr1_5/1 -> COMPErr/3  "<VINP_CANMsgValidZoneFrTHCM_flg>"
  COMPErr/1 -> VINP_COMPErr_enum/1  "VINP_COMPErr_enum"
  COMPErr/2 -> Terminator_5/1
  [BHAL_outputs] -> slr_VHAL_EACProtectEnable_enum/1
  slr_VHAL_EACProtectEnable_enum/1 -> EACProtectEnable/1  "<VHAL_EACProtectEnable_enum>"
  True_VHAL_EACProtectEnable_enum/1 -> EACProtectEnable/2
  [inp_CanValid_bus] -> slr1_6/1
  slr1_6/1 -> EACProtectEnable/3  "<VINP_CANMsgValidZoneFrTHCM_flg>"
  EACProtectEnable/1 -> VINP_EACProtectEnable_enum/1  "VINP_EACProtectEnable_enum"
  EACProtectEnable/2 -> Terminator_6/1
  [BHAL_outputs] -> slr_VHAL_EWP3Err_enum/1
  slr_VHAL_EWP3Err_enum/1 -> EWP3Err/1  "<VHAL_EWP3Err_enum>"
  True_VHAL_EWP3Err_enum/1 -> EWP3Err/2
  [inp_CanValid_bus] -> slr1_7/1
  slr1_7/1 -> EWP3Err/3  "<VINP_CANMsgValidZoneFrTHCM_flg>"
  EWP3Err/1 -> VINP_EWP3Err_enum/1  "VINP_EWP3Err_enum"
  EWP3Err/2 -> Terminator_7/1
  [BHAL_outputs] -> slr_VHAL_EXV1Err_enum/1
  slr_VHAL_EXV1Err_enum/1 -> EXV1Err/1  "<VHAL_EXV1Err_enum>"
  True_VHAL_EXV1Err_enum/1 -> EXV1Err/2
  [inp_CanValid_bus] -> slr1_8/1
  slr1_8/1 -> EXV1Err/3  "<VINP_CANMsgValidZoneFrTHCM_flg>"
  EXV1Err/1 -> VINP_EXV1Err_enum/1  "VINP_EXV1Err_enum"
  EXV1Err/2 -> Terminator_8/1
  [BHAL_outputs] -> slr_VHAL_EXV2Err_enum/1
  slr_VHAL_EXV2Err_enum/1 -> EXV2Err/1  "<VHAL_EXV2Err_enum>"
  True_VHAL_EXV2Err_enum/1 -> EXV2Err/2
  [inp_CanValid_bus] -> slr1_9/1
  slr1_9/1 -> EXV2Err/3  "<VINP_CANMsgValidZoneFrTHCM_flg>"
  EXV2Err/1 -> VINP_EXV2Err_enum/1  "VINP_EXV2Err_enum"
  EXV2Err/2 -> Terminator_9/1
  [BHAL_outputs] -> slr_VHAL_FanErr_enum/1
  slr_VHAL_FanErr_enum/1 -> FanErr/1  "<VHAL_FanErr_enum>"
  True_VHAL_FanErr_enum/1 -> FanErr/2
  [inp_CanValid_bus] -> slr1_10/1
  slr1_10/1 -> FanErr/3  "<VINP_CANMsgValidZoneFrTHCM_flg>"
  FanErr/1 -> VINP_FanErr_enum/1  "VINP_FanErr_enum"
  FanErr/2 -> Terminator_10/1
  [BHAL_outputs] -> slr_VHAL_MotorInTemp_C/1
  slr_VHAL_MotorInTemp_C/1 -> MotorInTemp/1  "<VHAL_MotorInTemp_C>"
  True_VHAL_MotorInTemp_C/1 -> MotorInTemp/2
  [inp_CanValid_bus] -> slr1_11/1
  slr1_11/1 -> MotorInTemp/3  "<VINP_CANMsgValidZoneFrTHCM_flg>"
  MotorInTemp/1 -> VINP_MotorInTemp_C/1  "VINP_MotorInTemp_C"
  MotorInTemp/2 -> Terminator_11/1
  [BHAL_outputs] -> slr_VHAL_MotorInTempErr_enum/1
  slr_VHAL_MotorInTempErr_enum/1 -> MotorInTempErr/1  "<VHAL_MotorInTempErr_enum>"
  True_VHAL_MotorInTempErr_enum/1 -> MotorInTempErr/2
  [inp_CanValid_bus] -> slr1_12/1
  slr1_12/1 -> MotorInTempErr/3  "<VINP_CANMsgValidZoneFrTHCM_flg>"
  MotorInTempErr/1 -> VINP_MotorInTempErr_enum/1  "VINP_MotorInTempErr_enum"
  MotorInTempErr/2 -> Terminator_12/1
  [BHAL_outputs] -> slr_VHAL_MotorOutTemp_C/1
  slr_VHAL_MotorOutTemp_C/1 -> MotorOutTemp/1  "<VHAL_MotorOutTemp_C>"
  True_VHAL_MotorOutTemp_C/1 -> MotorOutTemp/2
  [inp_CanValid_bus] -> slr1_13/1
  slr1_13/1 -> MotorOutTemp/3  "<VINP_CANMsgValidZoneFrTHCM_flg>"
  MotorOutTemp/1 -> VINP_MotorOutTemp_C/1  "VINP_MotorOutTemp_C"
  MotorOutTemp/2 -> Terminator_13/1
  [BHAL_outputs] -> slr_VHAL_MotorOutTempErr_enum/1
  slr_VHAL_MotorOutTempErr_enum/1 -> MotorOutTempErr/1  "<VHAL_MotorOutTempErr_enum>"
  True_VHAL_MotorOutTempErr_enum/1 -> MotorOutTempErr/2
  [inp_CanValid_bus] -> slr1_14/1
  slr1_14/1 -> MotorOutTempErr/3  "<VINP_CANMsgValidZoneFrTHCM_flg>"
  MotorOutTempErr/1 -> VINP_MotorOutTempErr_enum/1  "VINP_MotorOutTempErr_enum"
  MotorOutTempErr/2 -> Terminator_14/1
  [BHAL_outputs] -> slr_VHAL_PTHighP_KPa/1
  slr_VHAL_PTHighP_KPa/1 -> PTHighP/1  "<VHAL_PTHighP_KPa>"
  True_VHAL_PTHighP_KPa/1 -> PTHighP/2
  [inp_CanValid_bus] -> slr1_15/1
  slr1_15/1 -> PTHighP/3  "<VINP_CANMsgValidZoneFrTHCM_flg>"
  PTHighP/1 -> VINP_PTHighP_KPa/1  "VINP_PTHighP_KPa"
  PTHighP/2 -> Terminator_15/1
  [BHAL_outputs] -> slr_VHAL_PTHighPErr_enum/1
  slr_VHAL_PTHighPErr_enum/1 -> PTHighPErr/1  "<VHAL_PTHighPErr_enum>"
  True_VHAL_PTHighPErr_enum/1 -> PTHighPErr/2
  [inp_CanValid_bus] -> slr1_16/1
  slr1_16/1 -> PTHighPErr/3  "<VINP_CANMsgValidZoneFrTHCM_flg>"
  PTHighPErr/1 -> VINP_PTHighPErr_enum/1  "VINP_PTHighPErr_enum"
  PTHighPErr/2 -> Terminator_16/1
  [BHAL_outputs] -> slr_VHAL_PTHighTact_C/1
  slr_VHAL_PTHighTact_C/1 -> PTHighTact/1  "<VHAL_PTHighTact_C>"
  True_VHAL_PTHighTact_C/1 -> PTHighTact/2
  [inp_CanValid_bus] -> slr1_17/1
  slr1_17/1 -> PTHighTact/3  "<VINP_CANMsgValidZoneFrTHCM_flg>"
  PTHighTact/1 -> VINP_PTHighTact_C/1  "VINP_PTHighTact_C"
  PTHighTact/2 -> Terminator_17/1
  [BHAL_outputs] -> slr_VHAL_PTHighTactErr_enum/1
  slr_VHAL_PTHighTactErr_enum/1 -> PTHighTactErr/1  "<VHAL_PTHighTactErr_enum>"
  True_VHAL_PTHighTactErr_enum/1 -> PTHighTactErr/2
  [inp_CanValid_bus] -> slr1_18/1
  slr1_18/1 -> PTHighTactErr/3  "<VINP_CANMsgValidZoneFrTHCM_flg>"
  PTHighTactErr/1 -> VINP_PTHighTactErr_enum/1  "VINP_PTHighTactErr_enum"
  PTHighTactErr/2 -> Terminator_18/1
  [BHAL_outputs] -> slr_VHAL_PTLowP1_KPa/1
  slr_VHAL_PTLowP1_KPa/1 -> PTLowP1/1  "<VHAL_PTLowP1_KPa>"
  True_VHAL_PTLowP1_KPa/1 -> PTLowP1/2
  [inp_CanValid_bus] -> slr1_19/1
  slr1_19/1 -> PTLowP1/3  "<VINP_CANMsgValidZoneFrTHCM_flg>"
  PTLowP1/1 -> VINP_PTLowP1_KPa/1  "VINP_PTLowP1_KPa"
  PTLowP1/2 -> Terminator_19/1
  [BHAL_outputs] -> slr_VHAL_PTLowP1Err_enum/1
  slr_VHAL_PTLowP1Err_enum/1 -> PTLowP1Err/1  "<VHAL_PTLowP1Err_enum>"
  True_VHAL_PTLowP1Err_enum/1 -> PTLowP1Err/2
  [inp_CanValid_bus] -> slr1_20/1
  slr1_20/1 -> PTLowP1Err/3  "<VINP_CANMsgValidZoneFrTHCM_flg>"
  PTLowP1Err/1 -> VINP_PTLowP1Err_enum/1  "VINP_PTLowP1Err_enum"
  PTLowP1Err/2 -> Terminator_20/1
  [BHAL_outputs] -> slr_VHAL_PTLowP2_KPa/1
  slr_VHAL_PTLowP2_KPa/1 -> PTLowP2/1  "<VHAL_PTLowP2_KPa>"
  True_VHAL_PTLowP2_KPa/1 -> PTLowP2/2
  [inp_CanValid_bus] -> slr1_21/1
  slr1_21/1 -> PTLowP2/3  "<VINP_CANMsgValidZoneFrTHCM_flg>"
  PTLowP2/1 -> VINP_PTLowP2_KPa/1  "VINP_PTLowP2_KPa"
  PTLowP2/2 -> Terminator_21/1
  [BHAL_outputs] -> slr_VHAL_PTLowP2Err_enum/1
  slr_VHAL_PTLowP2Err_enum/1 -> PTLowP2Err/1  "<VHAL_PTLowP2Err_enum>"
  True_VHAL_PTLowP2Err_enum/1 -> PTLowP2Err/2
  [inp_CanValid_bus] -> slr1_22/1
  slr1_22/1 -> PTLowP2Err/3  "<VINP_CANMsgValidZoneFrTHCM_flg>"
  PTLowP2Err/1 -> VINP_PTLowP2Err_enum/1  "VINP_PTLowP2Err_enum"
  PTLowP2Err/2 -> Terminator_22/1
  [BHAL_outputs] -> slr_VHAL_PTLowT1_C/1
  slr_VHAL_PTLowT1_C/1 -> PTLowT1/1  "<VHAL_PTLowT1_C>"
  True_VHAL_PTLowT1_C/1 -> PTLowT1/2
  [inp_CanValid_bus] -> slr1_23/1
  slr1_23/1 -> PTLowT1/3  "<VINP_CANMsgValidZoneFrTHCM_flg>"
  PTLowT1/1 -> VINP_PTLowT1_C/1  "VINP_PTLowT1_C"
  PTLowT1/2 -> Terminator_23/1
  [BHAL_outputs] -> slr_VHAL_PTLowT1Err_enum/1
  slr_VHAL_PTLowT1Err_enum/1 -> PTLowT1Err/1  "<VHAL_PTLowT1Err_enum>"
  True_VHAL_PTLowT1Err_enum/1 -> PTLowT1Err/2
  [inp_CanValid_bus] -> slr1_24/1
  slr1_24/1 -> PTLowT1Err/3  "<VINP_CANMsgValidZoneFrTHCM_flg>"
  PTLowT1Err/1 -> VINP_PTLowT1Err_enum/1  "VINP_PTLowT1Err_enum"
  PTLowT1Err/2 -> Terminator_24/1
  [BHAL_outputs] -> slr_VHAL_PTLowT2_C/1
  slr_VHAL_PTLowT2_C/1 -> PTLowT2/1  "<VHAL_PTLowT2_C>"
  True_VHAL_PTLowT2_C/1 -> PTLowT2/2
  [inp_CanValid_bus] -> slr1_25/1
  slr1_25/1 -> PTLowT2/3  "<VINP_CANMsgValidZoneFrTHCM_flg>"
  PTLowT2/1 -> VINP_PTLowT2_C/1  "VINP_PTLowT2_C"
  PTLowT2/2 -> Terminator_25/1
  [BHAL_outputs] -> slr_VHAL_PTLowT2Err_enum/1
  slr_VHAL_PTLowT2Err_enum/1 -> PTLowT2Err/1  "<VHAL_PTLowT2Err_enum>"
  True_VHAL_PTLowT2Err_enum/1 -> PTLowT2Err/2
  [inp_CanValid_bus] -> slr1_26/1
  slr1_26/1 -> PTLowT2Err/3  "<VINP_CANMsgValidZoneFrTHCM_flg>"
  PTLowT2Err/1 -> VINP_PTLowT2Err_enum/1  "VINP_PTLowT2Err_enum"
  PTLowT2Err/2 -> Terminator_26/1
  [BHAL_outputs] -> slr_VHAL_SOTXVErr_enum/1
  slr_VHAL_SOTXVErr_enum/1 -> SOTXVErr/1  "<VHAL_SOTXVErr_enum>"
  True_VHAL_SOTXVErr_enum/1 -> SOTXVErr/2
  [inp_CanValid_bus] -> slr1_27/1
  slr1_27/1 -> SOTXVErr/3  "<VINP_CANMsgValidZoneFrTHCM_flg>"
  SOTXVErr/1 -> VINP_SOTXVErr_enum/1  "VINP_SOTXVErr_enum"
  SOTXVErr/2 -> Terminator_27/1
  [BHAL_outputs] -> slr_VHAL_SOV1Err_enum/1
  slr_VHAL_SOV1Err_enum/1 -> SOV1Err/1  "<VHAL_SOV1Err_enum>"
  True_VHAL_SOV1Err_enum/1 -> SOV1Err/2
  [inp_CanValid_bus] -> slr1_28/1
  slr1_28/1 -> SOV1Err/3  "<VINP_CANMsgValidZoneFrTHCM_flg>"
  SOV1Err/1 -> VINP_SOV1Err_enum/1  "VINP_SOV1Err_enum"
  SOV1Err/2 -> Terminator_28/1
  [BHAL_outputs] -> slr_VHAL_SOV2Err_enum/1
  slr_VHAL_SOV2Err_enum/1 -> SOV2Err/1  "<VHAL_SOV2Err_enum>"
  True_VHAL_SOV2Err_enum/1 -> SOV2Err/2
  [inp_CanValid_bus] -> slr1_29/1
  slr1_29/1 -> SOV2Err/3  "<VINP_CANMsgValidZoneFrTHCM_flg>"
  SOV2Err/1 -> VINP_SOV2Err_enum/1  "VINP_SOV2Err_enum"
  SOV2Err/2 -> Terminator_29/1
  [BHAL_outputs] -> slr_VHAL_SOV3Err_enum/1
  slr_VHAL_SOV3Err_enum/1 -> SOV3Err/1  "<VHAL_SOV3Err_enum>"
  True_VHAL_SOV3Err_enum/1 -> SOV3Err/2
  [inp_CanValid_bus] -> slr1_30/1
  slr1_30/1 -> SOV3Err/3  "<VINP_CANMsgValidZoneFrTHCM_flg>"
  SOV3Err/1 -> VINP_SOV3Err_enum/1  "VINP_SOV3Err_enum"
  SOV3Err/2 -> Terminator_30/1
  [BHAL_outputs] -> slr_VHAL_Tamb_C/1
  slr_VHAL_Tamb_C/1 -> Tamb/1  "<VHAL_Tamb_C>"
  True_VHAL_Tamb_C/1 -> Tamb/2
  [inp_CanValid_bus] -> slr1_31/1
  slr1_31/1 -> Tamb/3  "<VINP_CANMsgValidZoneFrTHCM_flg>"
  Tamb/1 -> VINP_Tamb_C/1  "VINP_Tamb_C"
  Tamb/2 -> Terminator_31/1
  [BHAL_outputs] -> slr_VHAL_TambErr_enum/1
  slr_VHAL_TambErr_enum/1 -> TambErr/1  "<VHAL_TambErr_enum>"
  True_VHAL_TambErr_enum/1 -> TambErr/2
  [inp_CanValid_bus] -> slr1_32/1
  slr1_32/1 -> TambErr/3  "<VINP_CANMsgValidZoneFrTHCM_flg>"
  TambErr/1 -> VINP_TambErr_enum/1  "VINP_TambErr_enum"
  TambErr/2 -> Terminator_32/1
